simulink model "complex_addsub_blk"  (R2019a)
settings: Solver=VariableStepAuto  StartTime=0.0  StopTime=20  RelTol=1e-3
libraries: xbsIndex_r4 x6
settings Model: Creator=mybur  LastModifiedBy=mybur

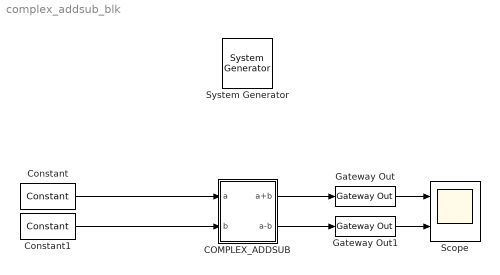
== system complex_addsub_blk ==
  " System Generator" : xbsIndex_r4/ System Generator  Tag=genX  xilinxfamily=kintex7  part=xc7k325t  speed=-3  package=fbg676  synthesis_tool=Vivado  clock_wrapper=Clock Enables  directory=./netlist  proj_type=Vivado  Synth_file=Vivado Synthesis Defaults  Impl_file=Vivado Implementation Defaults  testbench=off  simulink_period=1  sysclk_period=10  dcm_input_clock_period=10  incr_netlist=off  trim_vbits=Everywhere in SubSystem  dbl_ovrd=According to Block Masks  core_generation=According to Block Masks  run_coregen=off  deprecated_control=off  eval_field=0  block_type=sysgen
  COMPLEX_ADDSUB : Subsystem  mask(complex_addsub){bitwidth=10, add_latency=0}
      mask prompts: bitwidth "Bit Width"; add_latency "Add latency"
      mask help:
      | Adds and subtracts the complex inputs.
      | If a = w + ix, b = y + iz then
      | a+b = (w+y)/2 + i(x-z)/2 and
      | a-b = (x+z)/2 + i(y-w)/2
      mask init:
      | Simulink.Block.eval([gcb, '/complex_addsub']);
  Constant : xbsIndex_r4/Constant  const=181  gui_display_data_type=Fixed-point  arith_type=Unsigned  n_bits=8  bin_pt=0  preci_type=Single  exp_width=8  frac_width=24  explicit_period=on  period=1  equ=P=C  opselect=C  inp2=PCIN>>17  opr=+  inp1=P  carry=CIN  dbl_ovrd=off  block_type=constant
  Constant1 : xbsIndex_r4/Constant  const=87  gui_display_data_type=Fixed-point  arith_type=Unsigned  n_bits=8  bin_pt=0  preci_type=Single  exp_width=8  frac_width=24  explicit_period=on  period=1  equ=P=C  opselect=C  inp2=PCIN>>17  opr=+  inp1=P  carry=CIN  dbl_ovrd=off  block_type=constant
  Gateway Out : xbsIndex_r4/Gateway Out  inherit_from_input=off  hdl_port=on  rows=1  columns=1  UseAsDAC=off  DACChannel='1'  interface=None  automatic_assignment=on  address_offset=hex2dec('00')  intf_name=''  intf_description=''  timing_constraint=None  locs_specified=off  LOCs={}  io_standard={}  block_type=gatewayout
  Gateway Out1 : xbsIndex_r4/Gateway Out  inherit_from_input=off  hdl_port=on  rows=1  columns=1  UseAsDAC=off  DACChannel='1'  interface=None  automatic_assignment=on  address_offset=hex2dec('00')  intf_name=''  intf_description=''  timing_constraint=None  locs_specified=off  LOCs={}  io_standard={}  block_type=gatewayout
  Scope : Scope  NumInputPorts=2
  wires:
  Constant/1 -> COMPLEX_ADDSUB/1(a)
  Constant1/1 -> COMPLEX_ADDSUB/2(b)
  COMPLEX_ADDSUB/1(a+b) -> Gateway Out/1
  COMPLEX_ADDSUB/2(a-b) -> Gateway Out1/1
  Gateway Out/1 -> Scope/1
  Gateway Out1/1 -> Scope/2

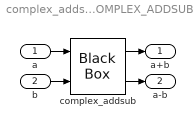
== system complex_addsub_blk/COMPLEX_ADDSUB ==
  a : Inport
  b : Inport  Port=2
  complex_addsub : xbsIndex_r4/Black Box  init_code=complex_addsub_config  sim_method=ISE Simulator  verbose=off  block_type=blackbox2
  a+b : Outport
  a-b : Outport  Port=2
  wires:
  b/1 -> complex_addsub/2
  complex_addsub/1 -> a+b/1
  a/1 -> complex_addsub/1
  complex_addsub/2 -> a-b/1
